simulink model "P8SIMULINK"  (R2024a)
settings: Solver=VariableStepAuto  StartTime=0.0  StopTime=10  RelTol=1e-3
InitFcn:
  | R=2;
  | Kt=0.01;
  | b=0.0012;
  | L=0.023;
  | Ke=0.01;
  | J=0.001;
settings Model: Creator=Becho  LastModifiedBy=Becho

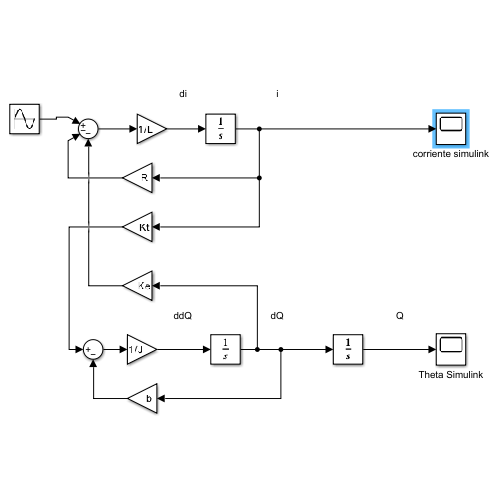
[thumbnail: Simulink's stored preview of the top-level diagram]
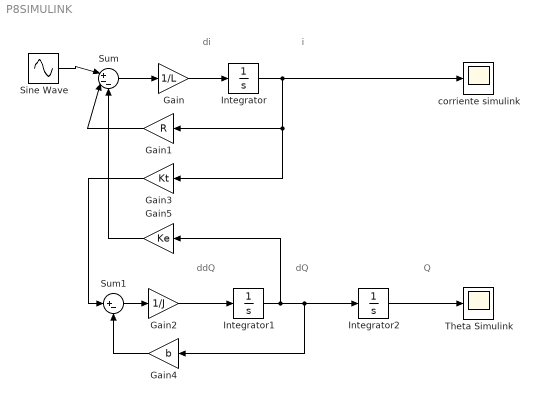
== system P8SIMULINK ==
  note: di
  note: i
  note: ddQ
  note: dQ
  note: Q
  Gain : Gain  Gain=1/L
  Gain1 : Gain  Gain=R
  Gain2 : Gain  Gain=1/J
  Gain3 : Gain  Gain=Kt
  Gain4 : Gain  Gain=b
  Gain5 : Gain  Gain=Ke
  Integrator : Integrator
  Integrator1 : Integrator
  Integrator2 : Integrator
  Sine Wave : Sin  Frequency=628.318530718  SampleTime=0
  Sum : Sum  Inputs=|+--
  Sum1 : Sum  Inputs=|+-
  Theta Simulink : Scope
  corriente simulink : Scope
  wires:
  Gain/1 -> Integrator/1
  Sum/1 -> Gain/1
  Integrator/1 -> corriente simulink/1, Gain3/1, Gain1/1
  Gain1/1 -> Sum/2
  Integrator1/1 -> Gain4/1, Integrator2/1, Gain5/1
  Gain2/1 -> Integrator1/1
  Sum1/1 -> Gain2/1
  Gain3/1 -> Sum1/1
  Gain4/1 -> Sum1/2
  Gain5/1 -> Sum/3
  Integrator2/1 -> Theta Simulink/1
  Sine Wave/1 -> Sum/1
